simulink model "hdlcoder_I2S_ssm2603"  (R2020b)
settings: Solver=FixedStepDiscrete  StartTime=0.0  StopTime=10000  RelTol=1e-3
InitFcn:
  | % Generate bit sequence of example I2S data
  | % BCLK period is 16 sample
  | % LRCLK period is 64 BCLK
  | i2s_data = fi([1e6:1e6:4e6], 0, 24, 0);
  | i2s_databits = str2num(i2s_data.bin(:));
  | i2s_dataseq = [];
  | i2s_bitselect = 1;
  | for ii_bclk = 1:32*4
  |     for jj_clk = 1:16
  |         if mod(ii_bclk, 32) == 1
  |             i2s_databit = 0;
  |         elseif mod(ii_bclk, 32) > 1 && mod(ii_bclk, 32) <=25
  |             i2s_databit = i2s_databits(i2s_bitselect);
  |             if jj_clk == 16
  |                 i2s_bitselect = i2s_bitselect + 1;
  |             end
  |         else
  |             i2s_databit = 0;
  |         end
  |         i2s_dataseq = [i2s_dataseq; i2s_databit];
  |     end
  | 
  | end
  | i2s_datasequence.time = [];
  | i2s_datasequence.signals.values = i2s_dataseq(:);
  | i2s_datasequence.signals.dimensions =1;
libraries: hdlsllib x5, simulink x1
settings Model: DataTypeOverride=Off  Creator=The MathWorks, Inc.  LastModifiedBy=amatsumo
settings DataIOCC: SaveOutput=off  SaveTime=off  ReturnWorkspaceOutputs=off
settings OptimizationCC: BlockReduction=off  ConditionallyExecuteInputs=off  DefaultParameterBehavior=Inlined
settings DebuggingCC: AlgebraicLoopMsg=error  SingleTaskRateTransMsg=error  StrictBusMsg=ErrorOnBusTreatedAsVector  ArithmeticOperatorsInVariantConditions=warning
settings HardwareCC: ProdBitPerPointer=32  ProdBitPerSizeT=32  ProdBitPerPtrDiffT=32  ProdLargestAtomicFloat=None  ProdIntDivRoundTo=Undefined  ProdEndianess=Unspecified  ProdWordSize=32  ProdHWDeviceType=ASIC/FPGA->ASIC/FPGA  ProdEqTarget=off
settings SFSimCC: SimUseLocalCustomCode=off  CustomCodeUndefinedFunction=UseInterfaceOnly
settings RTWCC: RTWUseLocalCustomCode=off
settings CodeAppCC: StateflowObjectComments=on
settings ConfigComp: CovMetricSettings=dswe

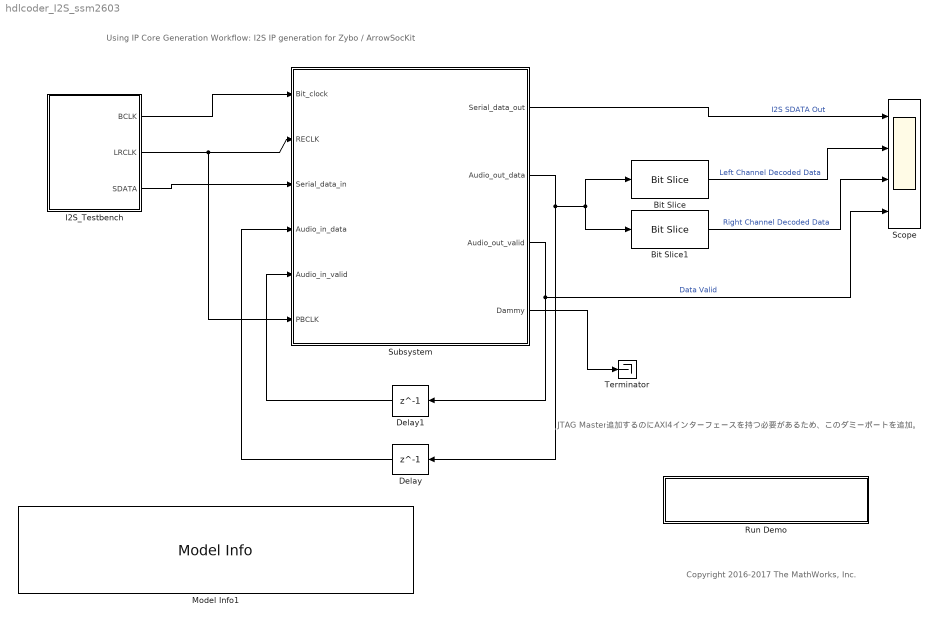
== system hdlcoder_I2S_ssm2603 ==
  note: JTAG Master追加するのにAXI4インターフェースを持つ必要があるため、このダミーポートを追加。
  note: Using IP Core Generation Workflow: I2S IP generation for Zybo / ArrowSocKit
  note: Copyright 2016-2017 The MathWorks, Inc.
  Bit Slice : hdlsllib/Logic and Bit Operations/Bit Slice  lidx=47  ridx=24
  Bit Slice1 : hdlsllib/Logic and Bit Operations/Bit Slice  lidx=23  ridx=0
  Delay : Delay  DelayLength=1
  Delay1 : Delay  DelayLength=1
  I2S_Testbench : Subsystem
  Model Info1 : simulink/Model-Wide Utilities/Model Info  Frame=on  DisplayStringWithTags=|  HorizontalTextAlignment=Left  LeftAlignmentValue=0.02
      | This example shows how to use HDL Workflow Advisor to 
      | generate a custom IP core for implementing I2S protocol 
      | 
      | In MATLAB, type the following:
      |   hdladvisor('hdlcoder_I2S_ssm2603/Subsystem')
  Run Demo : Subsystem
      settings: OpenFcn=hdladvisor([bdroot, '/led_counter'])
      mask Display: disp('Launch HDL Workflow Advisor')
  Scope : Scope  NumInputPorts=4
  Subsystem : Subsystem  TreatAsAtomicUnit=on
  Terminator : Terminator
  wires:
  Delay/1 -> Subsystem/4(Audio_in_data)
  Delay1/1 -> Subsystem/5("Audio_in_valid ")
  Subsystem/1("Serial_data_out ") -> Scope/1  "I2S SDATA Out"
  I2S_Testbench/1(BCLK) -> Subsystem/1(Bit_clock)
  I2S_Testbench/2(LRCLK) -> Subsystem/6(PBCLK), Subsystem/2(RECLK)
  I2S_Testbench/3(SDATA) -> Subsystem/3(Serial_data_in)
  Subsystem/3("Audio_out_valid ") -> Scope/4, Delay1/1  "Data Valid"
  Subsystem/2("Audio_out_data ") -> Bit Slice/1, Bit Slice1/1, Delay/1
  Bit Slice/1 -> Scope/2  "Left Channel Decoded Data"
  Bit Slice1/1 -> Scope/3  "Right Channel Decoded Data"
  Subsystem/4(Dammy) -> Terminator/1

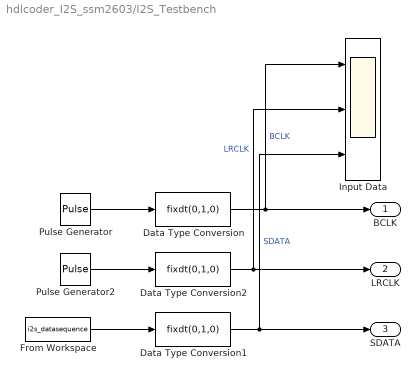
== system hdlcoder_I2S_ssm2603/I2S_Testbench ==
  Data Type Conversion : DataTypeConversion  OutDataTypeStr=fixdt(0,1,0)
  Data Type Conversion1 : DataTypeConversion  OutDataTypeStr=fixdt(0,1,0)
  Data Type Conversion2 : DataTypeConversion  OutDataTypeStr=fixdt(0,1,0)
  From Workspace : FromWorkspace  VariableName=i2s_datasequence  OutDataTypeStr=double  SampleTime=1  Interpolate=off  OutputAfterFinalValue=Cyclic repetition
  Input Data : Scope  NumInputPorts=3
  Pulse Generator : DiscretePulseGenerator  Period=16  PulseWidth=8  PhaseDelay=8
  Pulse Generator2 : DiscretePulseGenerator  Period=16*64  PulseWidth=8*64
  BCLK : Outport  VectorParamsAs1DForOutWhenUnconnected=off
  LRCLK : Outport  Port=2  VectorParamsAs1DForOutWhenUnconnected=off
  SDATA : Outport  Port=3  VectorParamsAs1DForOutWhenUnconnected=off
  wires:
  Data Type Conversion1/1 -> SDATA/1, Input Data/3  "SDATA"
  Pulse Generator2/1 -> Data Type Conversion2/1
  Pulse Generator/1 -> Data Type Conversion/1
  Data Type Conversion/1 -> BCLK/1, Input Data/1  "BCLK"
  Data Type Conversion2/1 -> LRCLK/1, Input Data/2  "LRCLK"
  From Workspace/1 -> Data Type Conversion1/1

== system hdlcoder_I2S_ssm2603/Run Demo ==

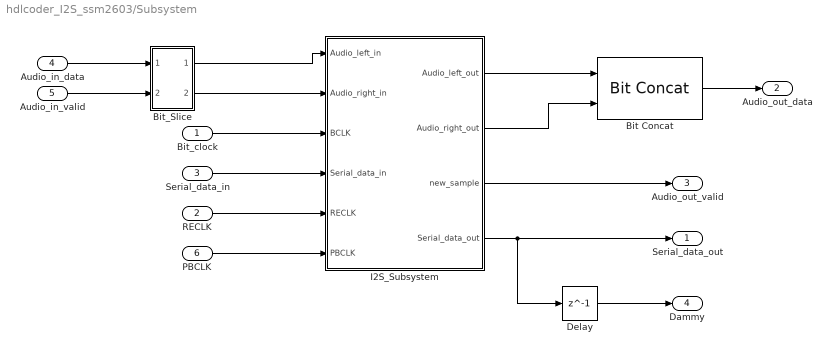
== system hdlcoder_I2S_ssm2603/Subsystem ==
  Bit_clock : Inport  OutDataTypeStr=fixdt(0, 1, 0)
  RECLK : Inport  Port=2  OutDataTypeStr=fixdt(0, 1, 0)
  Serial_data_in : Inport  Port=3  OutDataTypeStr=fixdt(0, 1, 0)
  Audio_in_data : Inport  Port=4  OutDataTypeStr=fixdt(0,48,0)
  "Audio_in_valid " : Inport  Port=5  OutDataTypeStr=boolean
  PBCLK : Inport  Port=6
  Bit Concat : hdlsllib/Logic and Bit Operations/Bit Concat  numInputs=2
      settings: SourceProductName=HDL Coder
  Bit_Slice : Subsystem
  Delay : Delay  DelayLength=1
  I2S_Subsystem : Subsystem
  "Serial_data_out " : Outport  OutDataTypeStr=fixdt(0, 1, 0)  VectorParamsAs1DForOutWhenUnconnected=off
  "Audio_out_data " : Outport  Port=2  OutDataTypeStr=fixdt(0,48,0)  VectorParamsAs1DForOutWhenUnconnected=off
  "Audio_out_valid " : Outport  Port=3  VectorParamsAs1DForOutWhenUnconnected=off
  Dammy : Outport  Port=4  OutDataTypeStr=fixdt(0, 1, 0)  VectorParamsAs1DForOutWhenUnconnected=off
  wires:
  I2S_Subsystem/3(new_sample) -> "Audio_out_valid "/1
  Bit_clock/1 -> I2S_Subsystem/3(BCLK)
  Serial_data_in/1 -> I2S_Subsystem/4(Serial_data_in)
  I2S_Subsystem/4(Serial_data_out) -> Delay/1, "Serial_data_out "/1
  I2S_Subsystem/1(Audio_left_out) -> Bit Concat/1
  I2S_Subsystem/2(Audio_right_out) -> Bit Concat/2
  Bit Concat/1 -> "Audio_out_data "/1
  Audio_in_data/1 -> Bit_Slice/1(In1)
  "Audio_in_valid "/1 -> Bit_Slice/2(In2)
  Bit_Slice/1(Out1) -> I2S_Subsystem/1(Audio_left_in)
  Bit_Slice/2(Out2) -> I2S_Subsystem/2(Audio_right_in)
  RECLK/1 -> I2S_Subsystem/5(RECLK)
  PBCLK/1 -> I2S_Subsystem/6(PBCLK)
  Delay/1 -> Dammy/1

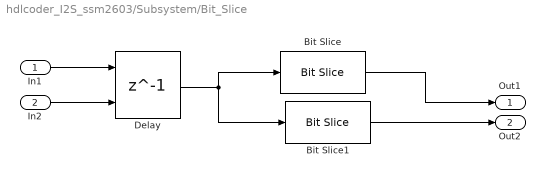
== system hdlcoder_I2S_ssm2603/Subsystem/Bit_Slice ==
  In1 : Inport
  In2 : Inport  Port=2
  Bit Slice : hdlsllib/Logic and Bit Operations/Bit Slice  lidx=47  ridx=24
  Bit Slice1 : hdlsllib/Logic and Bit Operations/Bit Slice  lidx=23  ridx=0
  Delay : Delay  DelayLength=1  ShowEnablePort=on
      settings: InputPortMap=u0,e6
  Out1 : Outport  VectorParamsAs1DForOutWhenUnconnected=off
  Out2 : Outport  Port=2  VectorParamsAs1DForOutWhenUnconnected=off
  wires:
  In2/1 -> Delay/2
  In1/1 -> Delay/1
  Bit Slice1/1 -> Out2/1
  Delay/1 -> Bit Slice1/1, Bit Slice/1
  Bit Slice/1 -> Out1/1

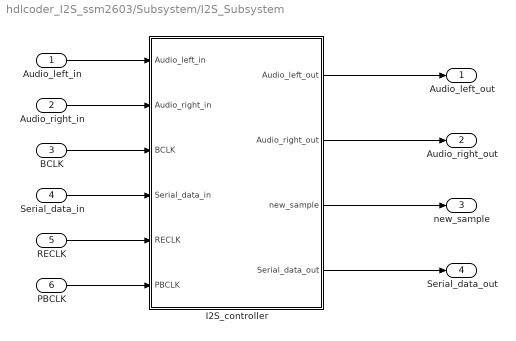
== system hdlcoder_I2S_ssm2603/Subsystem/I2S_Subsystem ==
  Audio_left_in : Inport
  Audio_right_in : Inport  Port=2
  BCLK : Inport  Port=3
  Serial_data_in : Inport  Port=4
  RECLK : Inport  Port=5
  PBCLK : Inport  Port=6
  I2S_controller : MATLAB Function  TreatAsAtomicUnit=on
  Audio_left_out : Outport  VectorParamsAs1DForOutWhenUnconnected=off
  Audio_right_out : Outport  Port=2  VectorParamsAs1DForOutWhenUnconnected=off
  new_sample : Outport  Port=3  VectorParamsAs1DForOutWhenUnconnected=off
  Serial_data_out : Outport  Port=4  VectorParamsAs1DForOutWhenUnconnected=off
  wires:
  Audio_left_in/1 -> I2S_controller/1(Audio_left_in)
  Audio_right_in/1 -> I2S_controller/2(Audio_right_in)
  BCLK/1 -> I2S_controller/3(BCLK)
  Serial_data_in/1 -> I2S_controller/4(Serial_data_in)
  RECLK/1 -> I2S_controller/5(RECLK)
  I2S_controller/1(Audio_left_out) -> Audio_left_out/1
  I2S_controller/2(Audio_right_out) -> Audio_right_out/1
  I2S_controller/3(new_sample) -> new_sample/1
  I2S_controller/4(Serial_data_out) -> Serial_data_out/1
  PBCLK/1 -> I2S_controller/6(PBCLK)

== matlab function hdlcoder_I2S_ssm2603/Subsystem/I2S_Subsystem/I2S_controller ==
  data: Audio_left_in input; Audio_left_out output; Audio_right_in input; BCLK input; Serial_data_in input; RECLK input; Audio_right_out output; new_sample output; Serial_data_out output; PBCLK input
function [Audio_left_out, Audio_right_out, new_sample, Serial_data_out] = Zybo_I2S_controller(Audio_left_in, Audio_right_in, BCLK, Serial_data_in, RECLK, PBCLK)

persistent BCLK_shiftreg sr_in_shiftreg sr_out_shiftreg RECLK_reg PBCLK_reg sr_in_reg Audio_left_out_reg Audio_right_out_reg Serial_data_out_reg
if isempty(BCLK_shiftreg)
    BCLK_shiftreg = fi(0, 0, 10, 0);
    sr_in_shiftreg = fi(0, 0, 127, 0);
    sr_out_shiftreg = fi(0, 0, 64, 0);
    RECLK_reg = fi(0, 0, 1, 0);
	PBCLK_reg = fi(0, 0, 1, 0);
    sr_in_reg = fi(0, 0, 1, 0);
    Audio_left_out_reg = fi(0, 0, 24, 0);
    Audio_right_out_reg = fi(0, 0, 24, 0);
    Serial_data_out_reg = fi(0, 0, 1, 0);
end

new_sample = false;

Audio_left_out = Audio_left_out_reg;
Audio_right_out = Audio_right_out_reg;
Serial_data_out = Serial_data_out_reg;

% detect rising edge of BCLK
% push the input data into input shift register
if bitsliceget(BCLK_shiftreg, 10, 9) == fi(2, 0, 2, 0)
    sr_in_shiftreg = bitconcat(bitsliceget(sr_in_shiftreg, 126, 1), sr_in_reg);
end

% if there is rising edge of BCLK 9 clock cycle ago, it menas it is near
% the falling edge of the BCLK
if bitsliceget(BCLK_shiftreg, 2, 1) == fi(2, 0, 2, 0)
    
    % push out output data from output shift register
    Serial_data_out_reg = bitsliceget(sr_out_shiftreg, 64, 64);
    
    % rising edge of RECLK
    if RECLK == fi(1, 0, 1, 0)&& RECLK_reg == fi(0, 0, 1, 0)
        Audio_left_out_reg = bitsliceget(sr_in_shiftreg, 127, 127-23);
        Audio_right_out_reg = bitsliceget(sr_in_shiftreg, 127-32, 127-23-32);
        new_sample = true;
    end	
    % rising edge of PBCLK
    if PBCLK == fi(1, 0, 1, 0)&& PBCLK_reg == fi(0, 0, 1, 0)
        sr_out_shiftreg = bitconcat(Audio_left_in, fi(0, 0, 8, 0), Audio_right_in, fi(0, 0, 8, 0));
    else
        sr_out_shiftreg = bitconcat(bitsliceget(sr_out_shiftreg, 63, 1), fi(0, 0, 1, 0));
    end
    RECLK_reg = RECLK;    
	PBCLK_reg = PBCLK;
end

% store BCLK in shift register
BCLK_shiftreg = bitconcat(BCLK, bitsliceget(BCLK_shiftreg, 10, 2));

sr_in_reg = Serial_data_in;
